simulink model "controlFuerza_2018a"  (R2018a)
settings: Solver=VariableStepAuto  StartTime=0.0  StopTime=0.1  RelTol=1e-3
values from neighbouring files (symbols this model uses):
  fd = [10*cos(pi/4), 10*sin(pi/4)]    [ctrl_fuerza.m]
  ke = diag([cos(pi/4)*Kenv, sin(pi/4)*Kenv])    [ctrl_fuerza.m]
  kpf = 0.01    [ctrl_fuerza.m]
  kvf = 2*sqrt(kpf)    [ctrl_fuerza.m]
  theta0_1 = -20.53*pi/180    (= -0.358316095434)    [ctrl_fuerza.m]
  theta0_2 = pi/4+abs(theta0_1)    [ctrl_fuerza.m]
libraries: roblocks x3, simulink x1
settings Model: Creator=Marcelo  LastModifiedBy=rochi
settings DataIOCC: ReturnWorkspaceOutputs=on
settings SFSimCC: SimUseLocalCustomCode=on
settings RTWCC: RTWUseLocalCustomCode=on

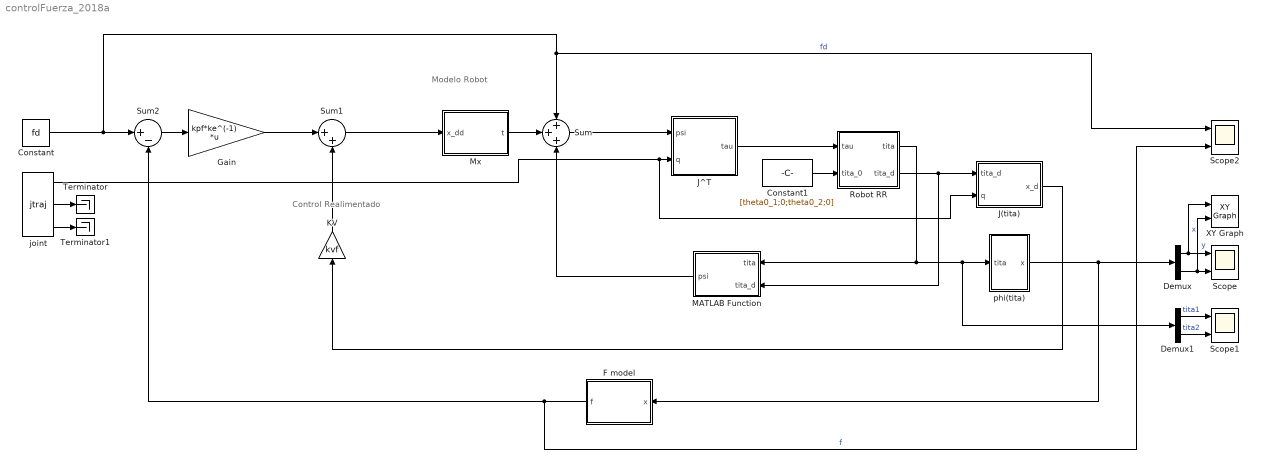
== system controlFuerza_2018a ==
  note: Control Realimentado
  note: Modelo Robot
  Constant : Constant  Value=fd
  Constant1 : Constant  Value=[theta0_1;0;theta0_2;0]
  Demux : Demux  Outputs=2
  Demux1 : Demux  Outputs=2
  "F model " : MATLAB Function  TreatAsAtomicUnit=on
  Gain : Gain  Gain=kpf*ke^(-1)  Multiplication=Matrix(K*u)
  J(tita) : MATLAB Function  TreatAsAtomicUnit=on
  J^T : MATLAB Function  TreatAsAtomicUnit=on
  KV : Gain  Gain=kvf
  MATLAB Function : MATLAB Function  TreatAsAtomicUnit=on
  Mx : MATLAB Function  TreatAsAtomicUnit=on
  Robot RR : Subsystem
  Scope : Scope  NumInputPorts=2
  Scope1 : Scope  NumInputPorts=2
  Scope2 : Scope  NumInputPorts=2
  Sum : Sum  Inputs=+++
  Sum1 : Sum  Inputs=|++
  Sum2 : Sum  Inputs=|+-
  Terminator : Terminator
  Terminator1 : Terminator
  XY Graph : simulink/Sinks/XY Graph  xmin=0  xmax=2  ymin=-1  ymax=2  st=-1
  joint : roblocks/Toolbox/jtraj  q0=[0 -pi/2]  qf=[pi/2 -pi/2]  tmax=10  ts=0.02
  phi(tita) : Subsystem
  wires:
  Robot RR/2(tita_d) -> J(tita)/1(tita_d), MATLAB Function/2(tita_d)
  KV/1 -> Sum1/2
  J(tita)/1(x_d) -> KV/1
  phi(tita)/1(x) -> "F model "/1(x), Demux/1
  Demux/1 -> XY Graph/1, Scope/1  "x"
  Demux/2 -> XY Graph/2, Scope/2  "y"
  Constant1/1 -> Robot RR/2(tita_0)
  Sum1/1 -> Mx/1(x_dd)
  Demux1/2 -> Scope1/2  "tita2"
  Demux1/1 -> Scope1/1  "tita1"
  J^T/1(tau) -> Robot RR/1(tau)
  Sum/1 -> J^T/1(psi)
  Robot RR/1(tita) -> Demux1/1, phi(tita)/1(tita), MATLAB Function/1(tita)
  MATLAB Function/1(psi) -> Sum/3
  Mx/1(t) -> Sum/2
  Constant/1 -> Sum2/1, Sum/1, Scope2/1  "fd"
  Gain/1 -> Sum1/1
  Sum2/1 -> Gain/1
  "F model "/1(f) -> Scope2/2, Sum2/2  "f"
  joint/1 -> J(tita)/2(q), J^T/2(q)
  joint/2 -> Terminator/1
  joint/3 -> Terminator1/1

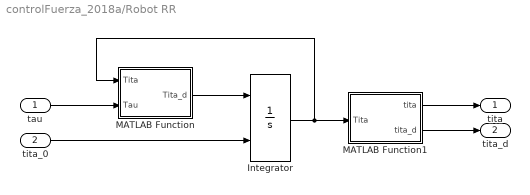
== system controlFuerza_2018a/Robot RR ==
  tau : Inport
  tita_0 : Inport  Port=2
  Integrator : Integrator  InitialConditionSource=external
  MATLAB Function : MATLAB Function  TreatAsAtomicUnit=on
  MATLAB Function1 : MATLAB Function  TreatAsAtomicUnit=on
  tita : Outport
  tita_d : Outport  Port=2
  wires:
  tau/1 -> MATLAB Function/2(Tau)
  MATLAB Function/1(Tita_d) -> Integrator/1
  tita_0/1 -> Integrator/2
  Integrator/1 -> MATLAB Function1/1(Tita), MATLAB Function/1(Tita)
  MATLAB Function1/1(tita) -> tita/1
  MATLAB Function1/2(tita_d) -> tita_d/1

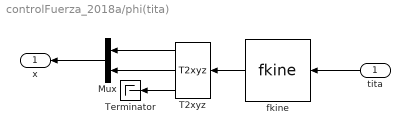
== system controlFuerza_2018a/phi(tita) ==
  tita : Inport
  Mux : Mux  Inputs=2
  T2xyz : roblocks/Toolbox/T2xyz
  Terminator : Terminator
  fkine : roblocks/Arm/fkine  robot=Robot
  x : Outport
  wires:
  T2xyz/2 -> Mux/2
  Mux/1 -> x/1
  fkine/1 -> T2xyz/1
  tita/1 -> fkine/1
  T2xyz/1 -> Mux/1
  T2xyz/3 -> Terminator/1

== matlab function controlFuerza_2018a/MATLAB Function ==
  data: tita input; psi output; tita_d input
function psi = f(tita,tita_d)

psi1 = tita_d(1);
psi2 = tita_d(2);

psi = [psi1;psi2];

== matlab function controlFuerza_2018a/J^T ==
  data: psi input; tau output; q input
function tau = fcn(psi,q)

th2 = q(2);
J = [sin(th2) 0; cos(th2)+1 1];

tau = (J')*psi;

== matlab function controlFuerza_2018a/Robot RR/MATLAB Function ==
  data: Tita input; Tita_d output; Tau input
function Tita_d = fcn(Tita,Tau)

titad1 = Tita(2);
titadd1 = Tau(1)-Tita(2);
titad2 = Tau(2);
titadd2 = 0;

Tita_d = [titad1;titadd1;titad2;titadd2];

== matlab function controlFuerza_2018a/Robot RR/MATLAB Function1 ==
  data: Tita input; tita output; tita_d output
function [tita,tita_d] = fcn(Tita)

tita = [Tita(1);Tita(3)];
tita_d = [Tita(2);Tita(4)];

== matlab function controlFuerza_2018a/F model  ==
  data: x input; f output
function f = fcn(x)
p1 = [0; 2];
p2 = [2; 0];

% checkeo de que lado de la pared esta el punto
% https://stackoverflow.com/questions/3838319/how-can-i-check-if-a-point-is-below-a-line-or-not
v1 = p2-p1;  % v1 = [2, -2] siempre
v2 = p2-x;   % v2 = [2-x, -y]
cross_prod = v1(1)*v2(2)-v1(2)*v2(1);
% ejemplo: si (x,y) = (0, 0), v2=[2, 0] y cross_prod=2*0+2*2=+4 > 0
% entonces el lado en el que estoy "adentro de la pared"
% es el que corresponde a cross(v1, v2) < 0
if cross_prod < 0
    K_env = 1e6; % 1000N/mm = 1e6N/m
    ke = diag([cos(pi/4)*K_env, sin(pi/4)*K_env]);
    % calculo del punto mas cercano a x sobre la recta ax+by+c=0
    % nuestra recta es x+y-2=0
    a = 1;
    b = 1;
    c = -2;
    x0 = x(1); y0 = x(2);
    xp1 = (b*(x0-a*y0)-a*c) / (a^2+b^2);
    xp2 = (a*(-b*x0+a*y0)-b*c) / (a^2+b^2);
    xp = [xp1; xp2];

    f = ke * (x - xp);
else
    f = [0; 0];
end

% 
% % distancia de un punto a una linea definida por dos puntos:
% % https://en.wikipedia.org/wiki/Distance_from_a_point_to_a_line
% 
% % esto podria simplificarse porque hay terminos que son 0, pero asi queda
% % generico para cualquier pared
% num = abs( (p2(2)-p1(2))*x(1) - (p2(1)-p1(1))*x(2)...
%     + p2(1)*p1(2) - p2(2)*p1(1) );
% % el denominador es la distancia entre los dos puntos que definen la linea
% den = dist(p1, p2);
% d = num/den;

== matlab function controlFuerza_2018a/J(tita) ==
  data: tita_d input; x_d output; q input
function x_d = fcn(tita_d,q)

th2 = q(2);
J = [sin(th2) 0; cos(th2)+1 1];

x_d = J*tita_d;

== matlab function controlFuerza_2018a/Mx ==
  data: x_dd input; t output
function t = fcn(x_dd)

t = [x_dd(1);0];
